simulink model "sm_common_gear_assembly_testrig"  (R2026a)
settings: Solver=ode45  MaxStep=0.01  EnableMultiTasking=on
undefined symbols (not defined in the file or in its folder): Local, Z
libraries: sm_lib x3, Multibody_Parts_Lib x2, nesl_utility x2
CloseFcn:
  | try,close(h1_sm_common_gear_assembly_testrig),end
  | clear h1_sm_common_gear_assembly_testrig
  | try,close(h2_sm_common_gear_assembly_testrig),end
  | clear h2_sm_common_gear_assembly_testrig
  | try,close(h3_sm_common_gear_assembly_testrig),end
  | clear h3_sm_common_gear_assembly_testrig
  | try,close(h4_sm_common_gear_assembly_testrig),end
  | clear h4_sm_common_gear_assembly_testrig
  | 
  | 
  | clear simlog_sm_common_gear_assembly_testrig
  | clear logsout_sm_common_gear_assembly_testrig
Description:
  | Common Gear Assembly Testrig
  | 
  | Copyright 2014-2026 The MathWorks, Inc.
settings Model: Creator=smiller  LastModifiedBy=smiller
settings DataIOCC: SignalLoggingName=logsout_sm_common_gear_assembly_testrig
settings DebuggingCC: UnderspecifiedInitializationDetection=Classic  PregeneratedLibrarySubsystemCodeDiagnostic=none
settings HardwareCC: ProdHWDeviceType=32-bit Generic
settings SimscapeCC: SimscapeNormalizeSystem=off  SimscapeNominalValues="[{\"value\":\"1\",\"unit\":\"A\"},{\"value\":\"1\",\"unit\":\"bar\"},{\"value\":\"1\",\"unit\":\"cm^2\"},{\"value\":\"1\",\"unit\":\"cm^3/s\"},{\"value\":\"1\",\"unit\":\"kJ/kg\"},{\"value\":\"1\",\"unit\":\"kW\"},{\"value\":\"1\",\"unit\":\"l\"},{\"value\":\"1\",\"unit\":\"N\"},{\"value\":\"1\",\"unit\":\"N*m\"},{\"value\":\"1\",\"unit\":\"V\"}]"  SimscapeLogSimulationStatistics=on  SimscapeLogName=simlog_sm_common_gear_assembly_testrig
settings ConfigurationSet: Description=SimMechanics 2G
settings ExplorerConfigSet: InternalSimMechanicsExplorerSettings="<ExplorerConfiguration><canonicalview>default</canonicalview><AnimationSetting><BasePlaybackSpeed>1.0</BasePlaybackSpeed><PlaybackSpeedFactor>1.0</PlaybackSpeedFactor></AnimationSetting><TilePanel><TileInfo><Tiles Columns=\"1\" Count=\"1\" Rows=\"1\"><Column Left=\"2\" Weight=\"1\"/><Column Left=\"655\"/><Row Top=\"2\" Weight=\"1\"/><Row Top=\"641\"/><Tile Height=\"1\" Width=\"1\" X=\"0\" Y=\"0\"/></Tiles></TileInfo><SceneInfo><SceneViewer><BGColor><R>1</R><G>1</G><B>1</B></BGColor><Camera><DoPerspective>off</DoPerspective><Position><X>0.48795763654664748</X><Y>0.21651936445992259</Y><Z>0.88163947123060693</Z></Position><Center><X>0.11172652849564876</X><Y>-0.03233641710704481</Y><Z>-0.01084075449736701</Z></Center><Up><X>-0.14306572804540199</X><Y>0.96730547632471442</Y><Z>-0.20940943849563221</Z></Up><ViewLimDist>1</ViewLimDist><YLim>0.21536772847175598</YLim><XLim>0.22015367799335053</XLim></Camera></SceneViewer></SceneInfo></TilePanel><MechEditorPanel><Cameras/><GfxPanelCameraMap/><VideoCreator><PlaybackSpeedRatio>1.0</PlaybackSpeedRatio><FrameRate>30</FrameRate><VideoFormat>Motion JPEG AVI</VideoFormat><FrameSize>auto</FrameSize></VideoCreator></MechEditorPanel></ExplorerConfiguration>"

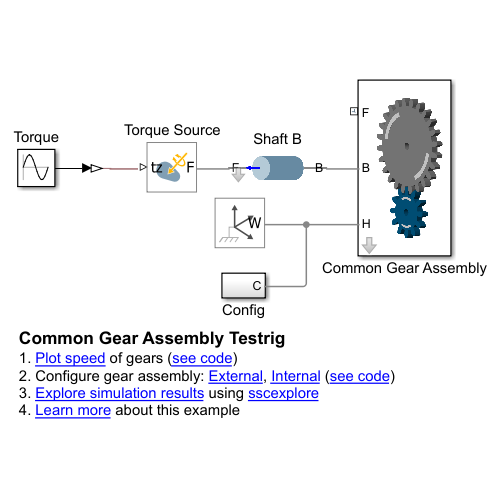
[thumbnail: Simulink's stored preview of the top-level diagram]
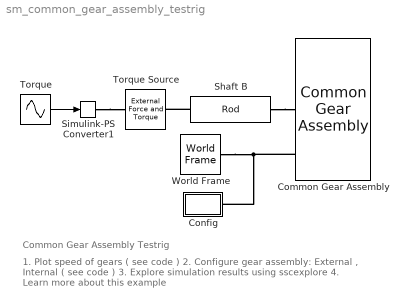
== system sm_common_gear_assembly_testrig ==
  note: Common Gear Assembly Testrig
  note: 1. Plot speed of gears ( see code )
      | 2. Configure gear assembly: External , Internal ( see code )
      | 3. Explore simulation results using sscexplore
      | 4. Learn more about this example
  Common Gear Assembly : Multibody_Parts_Lib/Gears/Assemblies/Common Gear Assembly  Tag=PublishSubsystem  b_gear_pd_asy=0.125  f_gear_pd_asy=0.25  b_gear_nt=12  f_gear_nt=24  b_gear_th=0.02  f_gear_th=0.02  f_popup_gear_type=External  b_gear_rh=0.01  f_gear_rht=0.01  b_gear_offset_angle=0  f_gear_offset_angle=360/24/2  b_gear_rho=7000  f_gear_rho=7000  b_gear_clr=[0.0 0.4 0.6]  f_gear_clr=[0.6 0.6 0.6]  b_gear_opc=1  f_gear_opc=1  popup_ad_dd_asy=Default  b_gear_ad=0.125/12  f_gear_ad=0.25/24  b_gear_dd=1.157*0.125/12  f_gear_dd=1.157*0.25/24  b_visc_frict_asy=0.01  f_visc_frict_asy=0.01  b_popup_markings=Two  f_popup_markings=Two  b_mark_radius_range=[0.6 0.7]  f_mark_radius_range=[0.7 0.8]  b_mark_angle_range=60  f_mark_angle_range=60  b_mark_color=[1 1 1]  f_mark_color=[1 1 1]
      settings: SourceProductName=Simscape Multibody Parts Library
  Config : Subsystem
  Shaft B : Multibody_Parts_Lib/Basic/Rod  rod_rad=0.01  rod_len=0.2  rod_rho=7000  rod_color=[0.0 0.4 0.6]  rod_opc=1  popup_zori=Local +Z  popup_markings=None  mark_radius_range=[0.5 1.01]  mark_length_range=1.005  mark_angle_range=30  mark_color=[1 1 1]
      settings: SourceProductName=Simscape Multibody Parts Library
  Simulink-PS Converter1 : nesl_utility/Simulink-PS Converter  PhysicalDomain=network_engine_domain  SubClassName=ps_input  LeftPortType=input  RightPortType=output  PseudoPeriodic=off  Frequencies=[]  NoiseDistribution=none  NoiseParameters=[]  Unit=1  AffineConversion=off  FilteringAndDerivatives=zero  SimscapeFilterOrder=1  InputFilterTimeConstant=0.001  UdotUserProvided=1
  Torque : Sin  Amplitude=10  Frequency=pi  Phase=pi/2  SampleTime=0
  Torque Source : sm_lib/Forces and Torques/External Force and Torque  EnableForceX=off  EnableForceY=off  EnableForceZ=off  EnableForce=off  ForceResolutionFrame=AttachedFrame  EnableTorqueX=off  EnableTorqueY=off  EnableTorqueZ=on  EnableTorque=off  TorqueResolutionFrame=AttachedFrame
  World Frame : sm_lib/Frames and Transforms/World Frame
  wires:
  Torque/1 -> Simulink-PS Converter1/1
  connections:
  Shaft B/LConn1 -- Common Gear Assembly/LConn2
  Simulink-PS Converter1/RConn1 -- Torque Source/LConn1
  World Frame/RConn1 -- Common Gear Assembly/LConn3 -- Config/RConn1
  Shaft B/RConn1 -- Torque Source/RConn1

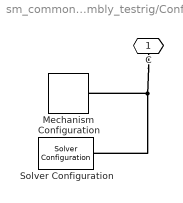
== system sm_common_gear_assembly_testrig/Config ==
  Mechanism Configuration : sm_lib/Utilities/Mechanism Configuration  UniformGravity=Constant  GravityVector=[0 -9.81 0]  GravityVectorUnits=m/s^2  LinearizationDelta=0.001  JointModeTransitionNonlinearIterations=2
  Solver Configuration : nesl_utility/Solver Configuration  PhysicalDomain=network_engine_domain  SubClassName=solver  LeftPortType=input  RightPortType=generic  Tones=[]  Harmonics=[]  SimulateNoise=off  Profile=off  UseLocalSampling=off  EnableSwitchedLinearOptims=on  FrequencyDomain=off  UseCCode=off  RelTol=0.001  AbsTol=1e-06  MinStep=1e-09  ToWorkspace=off  RevertToSquareIcSolve=off  NumHomotopyIterations=100  PhasorMode=off  PhasorModeNumHarmonics=1  ConsistencySolver=NEWTON_FTOL  CanonicalOrdering=UNORDERED  OptimizeIntermediates=UNOPTIMIZED  IndexReductionMethod=DerivativeReplacement  DoDC=off  ResidualTolerance=1e-09  ConsistencyTolSource=GLOBAL  ConsistencyAbsTol=0.001  ConsistencyRelTol=0.001  ConsistencyTolFactor=0.001  UseLocalSolver=off  LocalSolverChoice=NE_BACKWARD_EULER_ADVANCER  ResolveIndetEquations=on  FunctionEvalNumThread=1  LocalSolverSampleTime=0.001  DoFixedCost=off  MaxNonlinIter=3  MaxModeIter=2  ComputeImpulses=off  ImpulseIterations=2  LinearAlgebra=Sparse  LinearAlgebraNumThread=0  EquationFormulation=NE_TIME_EF  DelaysMemoryBudget=1024  AutomaticFiltering=on  FilteringTimeConstant=0.001  PartitionStorageMethod=AS_NEEDED  PartitionMemoryBudget=1024  PartitionMethod=FAST  MultibodyUseLocalSolver=off  MultibodyLocalSolverChoice=ODE1  MultibodyLocalSolverSampleTime=0.001
  C : PMIOPort  Side=Right
  connections:
  Mechanism Configuration/RConn1 -- C/RConn1 -- Solver Configuration/RConn1
